simulink model "Flight"  (R2022b)
settings: Solver=VariableStepAuto  StartTime=0.0  StopTime=10  RelTol=1e-3
libraries: simulink x1
settings Model: NumberOfSteps=10  Creator=Shloka Shetty  LastModifiedBy=aksha

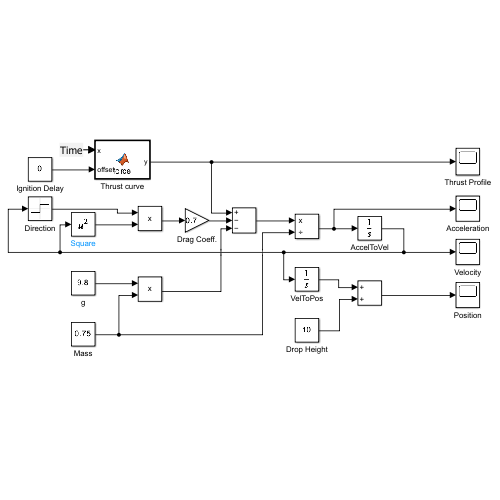
[thumbnail: Simulink's stored preview of the top-level diagram]
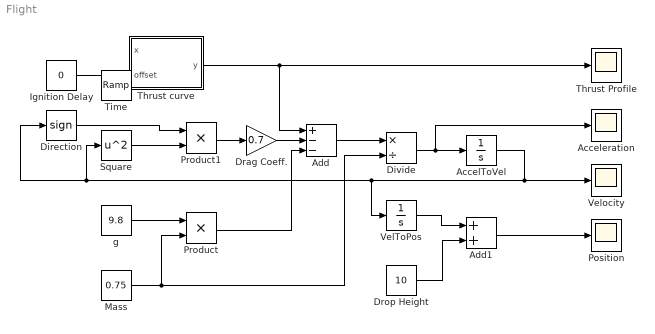
== system Flight ==
  AccelToVel : Integrator  ContinuousStateAttributes='acceleration'
  Acceleration : Scope
  Add : Sum  Inputs=+--
  Add1 : Sum
  Direction : Signum
  Divide : Product  Inputs=*/
  Drag Coeff. : Gain  Gain=0.7
  Drop Height : Constant  Value=10
  Ignition Delay : Constant  Value=0
  Mass : Constant  Value=0.75
  Position : Scope
  Product : Product
  Product1 : Product
  Square : Math  Operator=square
  Thrust Profile : Scope
  Thrust curve : MATLAB Function  TreatAsAtomicUnit=on
  VelToPos : Integrator  ContinuousStateAttributes='velocity'
  Velocity : Scope
  g : Constant  Value=9.8
  Time : simulink/Sources/Ramp  IOType=siggen  slope=1  start=0  InitialOutput=0
      settings: LibrarySourceBlock=simgens/Ramp
  wires:
  g/1 -> Product/1
  Mass/1 -> Divide/2, Product/2
  Product/1 -> Add/3
  Add/1 -> Divide/1
  Divide/1 -> Acceleration/1, AccelToVel/1
  VelToPos/1 -> Add1/1
  Add1/1 -> Position/1
  Drop Height/1 -> Add1/2
  Thrust curve/1(y) -> Add/1, Thrust Profile/1
  Ignition Delay/1 -> Thrust curve/2(offset)
  AccelToVel/1 -> Velocity/1, Direction/1, Square/1, VelToPos/1
  Drag Coeff./1 -> Add/2
  Product1/1 -> Drag Coeff./1
  Direction/1 -> Product1/1
  Square/1 -> Product1/2

== matlab function Flight/Thrust curve ==
  data: x input; y output; offset input
function y = force(x, offset)
    if x >= offset && x <= 0.25 + offset
        y = 120*(x-offset);
    elseif x >= 0.25 + offset && x <= 1 + offset
        %y = 10.0503 + 0.0847658/((x-offset)^3.94032);
        %y = -20213 + 20226.1/(x-offset)^0.0000294692;
        y = 9.9672 + 1311.23*exp(-14.5652*(x-offset));
    elseif x >= 1 + offset && x <= 2.8 + offset
        y = 10;
    else
        y = 0;
    end
end
